simulink model "dynamic_model_euler_with_s"  (R2021b)
settings: Solver=FixedStepAuto  StartTime=0.0  StopTime=simTime  FixedStep=sim_dt  RelTol=1e-3
undefined symbols (not defined in the file): d, g, J_platf, m_mass, m_platf, p, q0, roff, sim_dt, tau, umax, w0
libraries: matrix_library x1
settings Model: SimulationMode=accelerator  Creator=piszy  LastModifiedBy=krzysztof
settings SolverCC: ZeroCrossControl=DisableAll  AlgebraicLoopSolver=TrustRegion
settings DataIOCC: SaveOutput=off  SaveTime=off
settings OptimizationCC: BlockReduction=off  DefaultParameterBehavior=Inlined  BufferReuse=off
settings ModelReferenceCC: ModelReferenceNumInstancesAllowed=Single
settings SFSimCC: CustomCodeUndefinedFunction=UseInterfaceOnly
settings GRTTargetCC: CombineOutputUpdateFcns=off  MatFileLogging=off

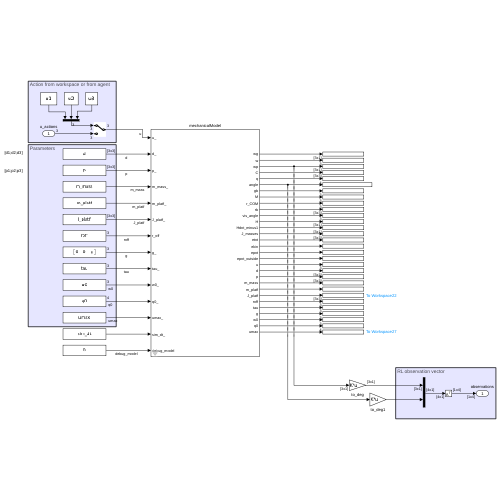
[thumbnail: Simulink's stored preview of the top-level diagram]
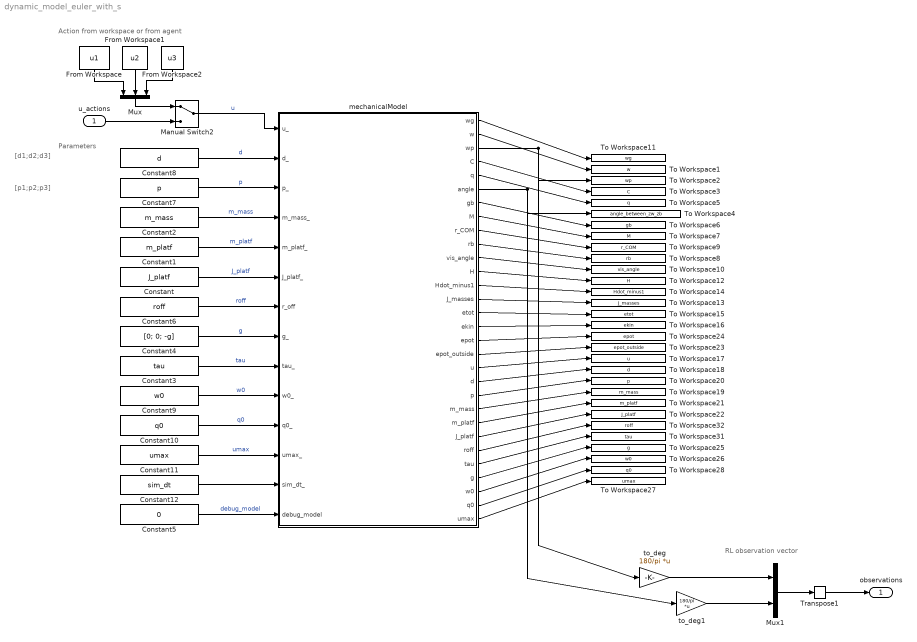
== system dynamic_model_euler_with_s ==
  note: Parameters
  note: Action from workspace or from agent
  note: RL observation vector
  note: [p1;p2;p3]
  note: [d1;d2;d3]
  u_actions : Inport  PortDimensions=[3]
  Constant : Constant  Value=J_platf
  Constant1 : Constant  Value=m_platf
  Constant10 : Constant  Value=q0
  Constant11 : Constant  Value=umax
  Constant12 : Constant  Value=sim_dt
  Constant2 : Constant  Value=m_mass
  Constant3 : Constant  Value=tau
  Constant4 : Constant  Value=[0; 0; -g]
  Constant5 : Constant  Value=0
  Constant6 : Constant  Value=roff
  Constant7 : Constant  Value=p
  Constant8 : Constant  Value=d
  Constant9 : Constant  Value=w0
  From Workspace : FromWorkspace  VariableName=u1
  From Workspace1 : FromWorkspace  VariableName=u2
  From Workspace2 : FromWorkspace  VariableName=u3
  Manual Switch2 : ManualSwitch
  Mux : Mux  Inputs=3
  Mux1 : Mux  Inputs=2
  To Workspace1 : ToWorkspace  VariableName=w  SampleTime=-1
  To Workspace10 : ToWorkspace  VariableName=vis_angle  SampleTime=-1
  To Workspace11 : ToWorkspace  VariableName=wg  SampleTime=-1
  To Workspace12 : ToWorkspace  VariableName=H  SampleTime=-1
  To Workspace13 : ToWorkspace  VariableName=J_masses  SampleTime=-1
  To Workspace14 : ToWorkspace  VariableName=Hdot_minus1  SampleTime=-1
  To Workspace15 : ToWorkspace  VariableName=etot  SampleTime=-1
  To Workspace16 : ToWorkspace  VariableName=ekin  SampleTime=-1
  To Workspace17 : ToWorkspace  VariableName=u  SampleTime=-1
  To Workspace18 : ToWorkspace  VariableName=d  SampleTime=-1
  To Workspace19 : ToWorkspace  VariableName=m_mass  SampleTime=-1
  To Workspace2 : ToWorkspace  VariableName=wp  SampleTime=-1
  To Workspace20 : ToWorkspace  VariableName=p  SampleTime=-1
  To Workspace21 : ToWorkspace  VariableName=m_platf  SampleTime=-1
  To Workspace22 : ToWorkspace  VariableName=J_platf  SampleTime=-1
  To Workspace23 : ToWorkspace  VariableName=epot_outside  SampleTime=-1
  To Workspace24 : ToWorkspace  VariableName=epot  SampleTime=-1
  To Workspace25 : ToWorkspace  VariableName=g  SampleTime=-1
  To Workspace26 : ToWorkspace  VariableName=w0  SampleTime=-1
  To Workspace27 : ToWorkspace  VariableName=umax  SampleTime=-1
  To Workspace28 : ToWorkspace  VariableName=q0  SampleTime=-1
  To Workspace3 : ToWorkspace  VariableName=C  SampleTime=-1
  To Workspace31 : ToWorkspace  VariableName=tau  SampleTime=-1
  To Workspace32 : ToWorkspace  VariableName=roff  SampleTime=-1
  To Workspace4 : ToWorkspace  VariableName=angle_between_zw_zb  SampleTime=-1
  To Workspace5 : ToWorkspace  VariableName=q  SampleTime=-1
  To Workspace6 : ToWorkspace  VariableName=gb  SampleTime=-1
  To Workspace7 : ToWorkspace  VariableName=M  SampleTime=-1
  To Workspace8 : ToWorkspace  VariableName=rb  SampleTime=-1
  To Workspace9 : ToWorkspace  VariableName=r_COM  SampleTime=-1
  Transpose1 : matrix_library/Transpose
      settings: SourceProductBaseCode=SL
  mechanicalModel : Subsystem
      mask help: Simulink:masks:GenSFuncDesc_MD
      mask Help: eval('feval(''rtwprivate'',''rtwhelpview'',''rtw_sfcn_block'')');
  to_deg : Gain  Gain=180/pi  Multiplication=Matrix(K*u)
  to_deg1 : Gain  Gain=180/pi  Multiplication=Matrix(K*u)
  observations : Outport
  wires:
  From Workspace/1 -> Mux/1
  From Workspace1/1 -> Mux/2
  From Workspace2/1 -> Mux/3
  Mux/1 -> Manual Switch2/1
  Manual Switch2/1 -> mechanicalModel/1(u_)  "u"
  u_actions/1 -> Manual Switch2/2
  Mux1/1 -> Transpose1/1
  Transpose1/1 -> observations/1
  Constant2/1 -> mechanicalModel/4(m_mass_)  "m_mass"
  Constant5/1 -> mechanicalModel/14(debug_model)  "debug_model"
  Constant8/1 -> mechanicalModel/2(d_)  "d"
  Constant7/1 -> mechanicalModel/3(p_)  "p"
  Constant1/1 -> mechanicalModel/5(m_platf_)  "m_platf"
  Constant3/1 -> mechanicalModel/9(tau_)  "tau"
  Constant6/1 -> mechanicalModel/7(r_off)  "roff"
  Constant4/1 -> mechanicalModel/8(g_)  "g"
  Constant/1 -> mechanicalModel/6(J_platf_)  "J_platf"
  mechanicalModel/6(angle) -> to_deg1/1, To Workspace4/1
  mechanicalModel/3(wp) -> to_deg/1, To Workspace2/1
  to_deg/1 -> Mux1/1
  to_deg1/1 -> Mux1/2
  Constant9/1 -> mechanicalModel/10(w0_)  "w0"
  Constant10/1 -> mechanicalModel/11(q0_)  "q0"
  Constant11/1 -> mechanicalModel/12(umax_)  "umax"
  Constant12/1 -> mechanicalModel/13(sim_dt_)
  mechanicalModel/1(wg) -> To Workspace11/1
  mechanicalModel/2(w) -> To Workspace1/1
  mechanicalModel/4(C) -> To Workspace3/1
  mechanicalModel/5(q) -> To Workspace5/1
  mechanicalModel/7(gb) -> To Workspace6/1
  mechanicalModel/8(M) -> To Workspace7/1
  mechanicalModel/9(r_COM) -> To Workspace9/1
  mechanicalModel/10(rb) -> To Workspace8/1
  mechanicalModel/11(vis_angle) -> To Workspace10/1
  mechanicalModel/12(H) -> To Workspace12/1
  mechanicalModel/13(Hdot_minus1) -> To Workspace14/1
  mechanicalModel/14(J_masses) -> To Workspace13/1
  mechanicalModel/15(etot) -> To Workspace15/1
  mechanicalModel/16(ekin) -> To Workspace16/1
  mechanicalModel/17(epot) -> To Workspace24/1
  mechanicalModel/18(epot_outside) -> To Workspace23/1
  mechanicalModel/19(u) -> To Workspace17/1
  mechanicalModel/20(d) -> To Workspace18/1
  mechanicalModel/21(p) -> To Workspace20/1
  mechanicalModel/22(m_mass) -> To Workspace19/1
  mechanicalModel/23(m_platf) -> To Workspace21/1
  mechanicalModel/24(J_platf) -> To Workspace22/1
  mechanicalModel/25(roff) -> To Workspace32/1
  mechanicalModel/26(tau) -> To Workspace31/1
  mechanicalModel/27(g) -> To Workspace25/1
  mechanicalModel/28(w0) -> To Workspace26/1
  mechanicalModel/29(q0) -> To Workspace28/1
  mechanicalModel/30(umax) -> To Workspace27/1

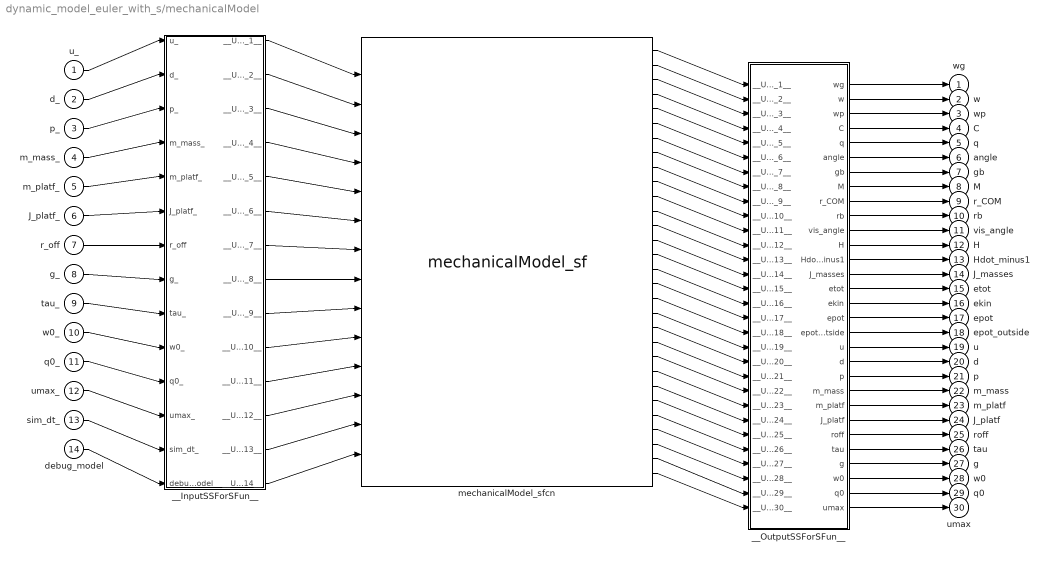
== system dynamic_model_euler_with_s/mechanicalModel ==
  u_ : Inport
  d_ : Inport  Port=2
  p_ : Inport  Port=3
  m_mass_ : Inport  Port=4
  m_platf_ : Inport  Port=5
  J_platf_ : Inport  Port=6
  r_off : Inport  Port=7
  g_ : Inport  Port=8
  tau_ : Inport  Port=9
  w0_ : Inport  Port=10
  q0_ : Inport  Port=11
  umax_ : Inport  Port=12
  sim_dt_ : Inport  Port=13
  debug_model : Inport  Port=14
  __InputSSForSFun__ : Subsystem
  __OutputSSForSFun__ : Subsystem
  mechanicalModel_sfcn : S-Function  FunctionName=mechanicalModel_sf  SFunctionModules=""  SFunctionDeploymentMode=off  EnableBusSupport=off  mask{rtw_sf_name=mechanicalModel_sf, showVar=off}
      mask prompts: rtw_sf_name "Simulink:masks:GenSFuncName_MP"; showVar "Simulink:masks:GenSFuncShowModuleList_MP"
      mask help: Simulink:masks:GenSFuncDesc_MD
      mask init:
      | displist = '';
      | if ~strcmp(get_param(gcb, 'FunctionName'), rtw_sf_name);
      |   set_param(gcb, 'FunctionName', rtw_sf_name);
      | end
      | % Check if we are generating code
      | rtw_mode = false;
      | if strcmpi(get_param(bdroot(gcb),'SimulationStatus'),'Initializing')
      | 	rtw_mode = strcmpi(get_param(bdroot(gcb),'BuildingRTWCode'),'on') && ...
      | 		~strcmpi(get_param(bdroot(gcb),'TargetStyle'),'SimulationTarget');
      | end
      | if showVar || rtw_mode
      | 	if exist('rtwsfunc') == 2 | exist('rtwsfunc') == 6
      | 		tmplist = rtwsfunc(rtw_sf_name,gcb);
      | 		tmplist = DAStudio.message('Simulink:masks:GenSFuncListOfModules_IC', tmplist);
      | 	elseif showVar
      | 		tmplist1 = DAStudio.message('Simulink:masks:GenSFuncListOfModules_IC', '');
      |         tmplist2 = DAStudio.message('Simulink:masks:GenSFuncNotLicensed_IC');
      |         tmplist = [tmplist1 tmplist2];
      |  	end
      | end
      | if showVar
      |   displist = tmplist;
      | end
      settings: CopyFcn=|
      | if ~strcmp(get_param(gcb,'Linkstatus'),'none') && ...
      | ~strcmp(get_param(gcb,'Linkstatus'),'implicit')
      |   set_param(gcb,'LinkStatus','none');
      | end
      mask Help: eval('feval(''rtwprivate'',''rtwhelpview'',''rtw_sfcn_block'')');
      mask Display:
      | port_label('input',1,'u_');
      | port_label('input',2,'d_');
      | port_label('input',3,'p_');
      | port_label('input',4,'m_mass_');
      | port_label('input',5,'m_platf_');
      | port_label('input',6,'J_platf_');
      | port_label('input',7,'r_off');
      | port_label('input',8,'g_');
      | port_label('input',9,'tau_');
      | port_label('input',10,'w0_');
      | port_label('input',11,'q0_');
      | port_label('input',12,'umax_');
      | port_label('input',13,'sim_dt_');
      | port_label('input',14,'debug_model');
      | port_label('output',1,'wg');
      | port_label('output',2,'w');
      | port_label('output',3,'wp');
      | port_label('output',4,'C');
      | port_label('output',5,'q');
      | port_label('output',6,'angle');
      | port_label('output',7,'gb');
      | port_label('output',8,'M');
      | port_label('output',9,'r_COM');
      | port_label('output',10,'rb');
      | port_label('output',11,'vis_angle');
      | port_label('output',12,'H');
      | port_label('output',13,'Hdot_minus1');
      | port_label('output',14,'J_masses');
      | port_label('output',15,'etot');
      | port_label('output',16,'ekin');
      | port_label('output',17,'epot');
      | port_label('output',18,'epot_outside');
      | port_label('output',19,'u');
      | port_label('output',20,'d');
      | port_label('output',21,'p');
      | port_label('output',22,'m_mass');
      | port_label('output',23,'m_platf');
      | port_label('output',24,'J_platf');
      | port_label('output',25,'roff');
      | port_label('output',26,'tau');
      | port_label('output',27,'g');
      | port_label('output',28,'w0');
      | port_label('output',29,'q0');
      | port_label('output',30,'umax');
  wg : Outport
  w : Outport  Port=2
  wp : Outport  Port=3
  C : Outport  Port=4
  q : Outport  Port=5
  angle : Outport  Port=6
  gb : Outport  Port=7
  M : Outport  Port=8
  r_COM : Outport  Port=9
  rb : Outport  Port=10
  vis_angle : Outport  Port=11
  H : Outport  Port=12
  Hdot_minus1 : Outport  Port=13
  J_masses : Outport  Port=14
  etot : Outport  Port=15
  ekin : Outport  Port=16
  epot : Outport  Port=17
  epot_outside : Outport  Port=18
  u : Outport  Port=19
  d : Outport  Port=20
  p : Outport  Port=21
  m_mass : Outport  Port=22
  m_platf : Outport  Port=23
  J_platf : Outport  Port=24
  roff : Outport  Port=25
  tau : Outport  Port=26
  g : Outport  Port=27
  w0 : Outport  Port=28
  q0 : Outport  Port=29
  umax : Outport  Port=30
  wires:
  __OutputSSForSFun__/30(umax) -> umax/1
  __OutputSSForSFun__/29(q0) -> q0/1
  __OutputSSForSFun__/28(w0) -> w0/1
  __OutputSSForSFun__/27(g) -> g/1
  __OutputSSForSFun__/26(tau) -> tau/1
  __OutputSSForSFun__/25(roff) -> roff/1
  __OutputSSForSFun__/24(J_platf) -> J_platf/1
  __OutputSSForSFun__/23(m_platf) -> m_platf/1
  __OutputSSForSFun__/22(m_mass) -> m_mass/1
  __OutputSSForSFun__/21(p) -> p/1
  __OutputSSForSFun__/20(d) -> d/1
  __OutputSSForSFun__/19(u) -> u/1
  __OutputSSForSFun__/18(epot_outside) -> epot_outside/1
  __OutputSSForSFun__/17(epot) -> epot/1
  __OutputSSForSFun__/16(ekin) -> ekin/1
  __OutputSSForSFun__/15(etot) -> etot/1
  __OutputSSForSFun__/14(J_masses) -> J_masses/1
  __OutputSSForSFun__/13(Hdot_minus1) -> Hdot_minus1/1
  __OutputSSForSFun__/12(H) -> H/1
  __OutputSSForSFun__/11(vis_angle) -> vis_angle/1
  __OutputSSForSFun__/10(rb) -> rb/1
  __OutputSSForSFun__/9(r_COM) -> r_COM/1
  __OutputSSForSFun__/8(M) -> M/1
  __OutputSSForSFun__/7(gb) -> gb/1
  __OutputSSForSFun__/6(angle) -> angle/1
  __OutputSSForSFun__/5(q) -> q/1
  __OutputSSForSFun__/4(C) -> C/1
  __OutputSSForSFun__/3(wp) -> wp/1
  __OutputSSForSFun__/2(w) -> w/1
  __OutputSSForSFun__/1(wg) -> wg/1
  mechanicalModel_sfcn/30 -> __OutputSSForSFun__/30(__UniqueInportName__30__)
  mechanicalModel_sfcn/29 -> __OutputSSForSFun__/29(__UniqueInportName__29__)
  mechanicalModel_sfcn/28 -> __OutputSSForSFun__/28(__UniqueInportName__28__)
  mechanicalModel_sfcn/27 -> __OutputSSForSFun__/27(__UniqueInportName__27__)
  mechanicalModel_sfcn/26 -> __OutputSSForSFun__/26(__UniqueInportName__26__)
  mechanicalModel_sfcn/25 -> __OutputSSForSFun__/25(__UniqueInportName__25__)
  mechanicalModel_sfcn/24 -> __OutputSSForSFun__/24(__UniqueInportName__24__)
  mechanicalModel_sfcn/23 -> __OutputSSForSFun__/23(__UniqueInportName__23__)
  mechanicalModel_sfcn/22 -> __OutputSSForSFun__/22(__UniqueInportName__22__)
  mechanicalModel_sfcn/21 -> __OutputSSForSFun__/21(__UniqueInportName__21__)
  mechanicalModel_sfcn/20 -> __OutputSSForSFun__/20(__UniqueInportName__20__)
  mechanicalModel_sfcn/19 -> __OutputSSForSFun__/19(__UniqueInportName__19__)
  mechanicalModel_sfcn/18 -> __OutputSSForSFun__/18(__UniqueInportName__18__)
  mechanicalModel_sfcn/17 -> __OutputSSForSFun__/17(__UniqueInportName__17__)
  mechanicalModel_sfcn/16 -> __OutputSSForSFun__/16(__UniqueInportName__16__)
  mechanicalModel_sfcn/15 -> __OutputSSForSFun__/15(__UniqueInportName__15__)
  mechanicalModel_sfcn/14 -> __OutputSSForSFun__/14(__UniqueInportName__14__)
  mechanicalModel_sfcn/13 -> __OutputSSForSFun__/13(__UniqueInportName__13__)
  mechanicalModel_sfcn/12 -> __OutputSSForSFun__/12(__UniqueInportName__12__)
  mechanicalModel_sfcn/11 -> __OutputSSForSFun__/11(__UniqueInportName__11__)
  mechanicalModel_sfcn/10 -> __OutputSSForSFun__/10(__UniqueInportName__10__)
  mechanicalModel_sfcn/9 -> __OutputSSForSFun__/9(__UniqueInportName__9__)
  mechanicalModel_sfcn/8 -> __OutputSSForSFun__/8(__UniqueInportName__8__)
  mechanicalModel_sfcn/7 -> __OutputSSForSFun__/7(__UniqueInportName__7__)
  mechanicalModel_sfcn/6 -> __OutputSSForSFun__/6(__UniqueInportName__6__)
  mechanicalModel_sfcn/5 -> __OutputSSForSFun__/5(__UniqueInportName__5__)
  mechanicalModel_sfcn/4 -> __OutputSSForSFun__/4(__UniqueInportName__4__)
  mechanicalModel_sfcn/3 -> __OutputSSForSFun__/3(__UniqueInportName__3__)
  mechanicalModel_sfcn/2 -> __OutputSSForSFun__/2(__UniqueInportName__2__)
  mechanicalModel_sfcn/1 -> __OutputSSForSFun__/1(__UniqueInportName__1__)
  __InputSSForSFun__/14(__UniqueOutportName__14__) -> mechanicalModel_sfcn/14
  __InputSSForSFun__/13(__UniqueOutportName__13__) -> mechanicalModel_sfcn/13
  __InputSSForSFun__/12(__UniqueOutportName__12__) -> mechanicalModel_sfcn/12
  __InputSSForSFun__/11(__UniqueOutportName__11__) -> mechanicalModel_sfcn/11
  __InputSSForSFun__/10(__UniqueOutportName__10__) -> mechanicalModel_sfcn/10
  __InputSSForSFun__/9(__UniqueOutportName__9__) -> mechanicalModel_sfcn/9
  __InputSSForSFun__/8(__UniqueOutportName__8__) -> mechanicalModel_sfcn/8
  __InputSSForSFun__/7(__UniqueOutportName__7__) -> mechanicalModel_sfcn/7
  __InputSSForSFun__/6(__UniqueOutportName__6__) -> mechanicalModel_sfcn/6
  __InputSSForSFun__/5(__UniqueOutportName__5__) -> mechanicalModel_sfcn/5
  __InputSSForSFun__/4(__UniqueOutportName__4__) -> mechanicalModel_sfcn/4
  __InputSSForSFun__/3(__UniqueOutportName__3__) -> mechanicalModel_sfcn/3
  __InputSSForSFun__/2(__UniqueOutportName__2__) -> mechanicalModel_sfcn/2
  __InputSSForSFun__/1(__UniqueOutportName__1__) -> mechanicalModel_sfcn/1
  debug_model/1 -> __InputSSForSFun__/14(debug_model)
  sim_dt_/1 -> __InputSSForSFun__/13(sim_dt_)
  umax_/1 -> __InputSSForSFun__/12(umax_)
  q0_/1 -> __InputSSForSFun__/11(q0_)
  w0_/1 -> __InputSSForSFun__/10(w0_)
  tau_/1 -> __InputSSForSFun__/9(tau_)
  g_/1 -> __InputSSForSFun__/8(g_)
  r_off/1 -> __InputSSForSFun__/7(r_off)
  J_platf_/1 -> __InputSSForSFun__/6(J_platf_)
  m_platf_/1 -> __InputSSForSFun__/5(m_platf_)
  m_mass_/1 -> __InputSSForSFun__/4(m_mass_)
  p_/1 -> __InputSSForSFun__/3(p_)
  d_/1 -> __InputSSForSFun__/2(d_)
  u_/1 -> __InputSSForSFun__/1(u_)

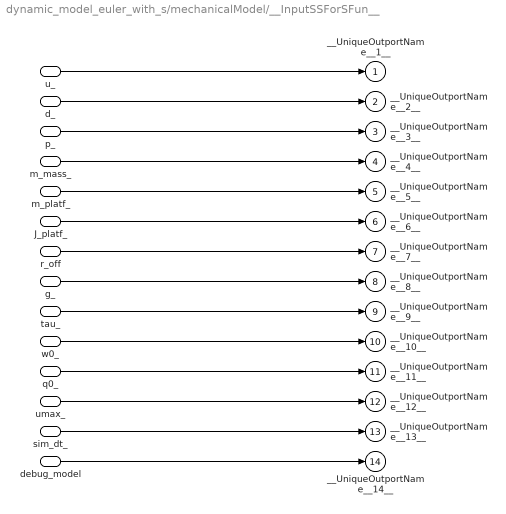
== system dynamic_model_euler_with_s/mechanicalModel/__InputSSForSFun__ ==
  u_ : Inport
  d_ : Inport  Port=2
  p_ : Inport  Port=3
  m_mass_ : Inport  Port=4
  m_platf_ : Inport  Port=5
  J_platf_ : Inport  Port=6
  r_off : Inport  Port=7
  g_ : Inport  Port=8
  tau_ : Inport  Port=9
  w0_ : Inport  Port=10
  q0_ : Inport  Port=11
  umax_ : Inport  Port=12
  sim_dt_ : Inport  Port=13
  debug_model : Inport  Port=14
  __UniqueOutportName__1__ : Outport
  __UniqueOutportName__2__ : Outport  Port=2
  __UniqueOutportName__3__ : Outport  Port=3
  __UniqueOutportName__4__ : Outport  Port=4
  __UniqueOutportName__5__ : Outport  Port=5
  __UniqueOutportName__6__ : Outport  Port=6
  __UniqueOutportName__7__ : Outport  Port=7
  __UniqueOutportName__8__ : Outport  Port=8
  __UniqueOutportName__9__ : Outport  Port=9
  __UniqueOutportName__10__ : Outport  Port=10
  __UniqueOutportName__11__ : Outport  Port=11
  __UniqueOutportName__12__ : Outport  Port=12
  __UniqueOutportName__13__ : Outport  Port=13
  __UniqueOutportName__14__ : Outport  Port=14
  wires:
  debug_model/1 -> __UniqueOutportName__14__/1
  sim_dt_/1 -> __UniqueOutportName__13__/1
  umax_/1 -> __UniqueOutportName__12__/1
  q0_/1 -> __UniqueOutportName__11__/1
  w0_/1 -> __UniqueOutportName__10__/1
  tau_/1 -> __UniqueOutportName__9__/1
  g_/1 -> __UniqueOutportName__8__/1
  r_off/1 -> __UniqueOutportName__7__/1
  J_platf_/1 -> __UniqueOutportName__6__/1
  m_platf_/1 -> __UniqueOutportName__5__/1
  m_mass_/1 -> __UniqueOutportName__4__/1
  p_/1 -> __UniqueOutportName__3__/1
  d_/1 -> __UniqueOutportName__2__/1
  u_/1 -> __UniqueOutportName__1__/1

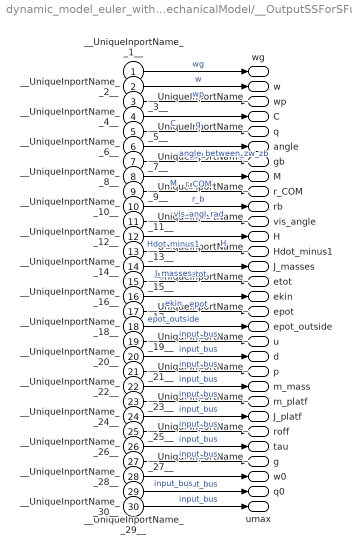
== system dynamic_model_euler_with_s/mechanicalModel/__OutputSSForSFun__ ==
  __UniqueInportName__1__ : Inport
  __UniqueInportName__2__ : Inport  Port=2
  __UniqueInportName__3__ : Inport  Port=3
  __UniqueInportName__4__ : Inport  Port=4
  __UniqueInportName__5__ : Inport  Port=5
  __UniqueInportName__6__ : Inport  Port=6
  __UniqueInportName__7__ : Inport  Port=7
  __UniqueInportName__8__ : Inport  Port=8
  __UniqueInportName__9__ : Inport  Port=9
  __UniqueInportName__10__ : Inport  Port=10
  __UniqueInportName__11__ : Inport  Port=11
  __UniqueInportName__12__ : Inport  Port=12
  __UniqueInportName__13__ : Inport  Port=13
  __UniqueInportName__14__ : Inport  Port=14
  __UniqueInportName__15__ : Inport  Port=15
  __UniqueInportName__16__ : Inport  Port=16
  __UniqueInportName__17__ : Inport  Port=17
  __UniqueInportName__18__ : Inport  Port=18
  __UniqueInportName__19__ : Inport  Port=19
  __UniqueInportName__20__ : Inport  Port=20
  __UniqueInportName__21__ : Inport  Port=21
  __UniqueInportName__22__ : Inport  Port=22
  __UniqueInportName__23__ : Inport  Port=23
  __UniqueInportName__24__ : Inport  Port=24
  __UniqueInportName__25__ : Inport  Port=25
  __UniqueInportName__26__ : Inport  Port=26
  __UniqueInportName__27__ : Inport  Port=27
  __UniqueInportName__28__ : Inport  Port=28
  __UniqueInportName__29__ : Inport  Port=29
  __UniqueInportName__30__ : Inport  Port=30
  wg : Outport
  w : Outport  Port=2
  wp : Outport  Port=3
  C : Outport  Port=4
  q : Outport  Port=5
  angle : Outport  Port=6
  gb : Outport  Port=7
  M : Outport  Port=8
  r_COM : Outport  Port=9
  rb : Outport  Port=10
  vis_angle : Outport  Port=11
  H : Outport  Port=12
  Hdot_minus1 : Outport  Port=13
  J_masses : Outport  Port=14
  etot : Outport  Port=15
  ekin : Outport  Port=16
  epot : Outport  Port=17
  epot_outside : Outport  Port=18
  u : Outport  Port=19
  d : Outport  Port=20
  p : Outport  Port=21
  m_mass : Outport  Port=22
  m_platf : Outport  Port=23
  J_platf : Outport  Port=24
  roff : Outport  Port=25
  tau : Outport  Port=26
  g : Outport  Port=27
  w0 : Outport  Port=28
  q0 : Outport  Port=29
  umax : Outport  Port=30
  wires:
  __UniqueInportName__30__/1 -> umax/1  "input_bus"
  __UniqueInportName__29__/1 -> q0/1  "input_bus"
  __UniqueInportName__28__/1 -> w0/1  "input_bus"
  __UniqueInportName__27__/1 -> g/1  "input_bus"
  __UniqueInportName__26__/1 -> tau/1  "input_bus"
  __UniqueInportName__25__/1 -> roff/1  "input_bus"
  __UniqueInportName__24__/1 -> J_platf/1  "input_bus"
  __UniqueInportName__23__/1 -> m_platf/1  "input_bus"
  __UniqueInportName__22__/1 -> m_mass/1  "input_bus"
  __UniqueInportName__21__/1 -> p/1  "input_bus"
  __UniqueInportName__20__/1 -> d/1  "input_bus"
  __UniqueInportName__19__/1 -> u/1  "input_bus"
  __UniqueInportName__18__/1 -> epot_outside/1  "epot_outside"
  __UniqueInportName__17__/1 -> epot/1  "epot"
  __UniqueInportName__16__/1 -> ekin/1  "ekin"
  __UniqueInportName__15__/1 -> etot/1  "etot"
  __UniqueInportName__14__/1 -> J_masses/1  "J_masses"
  __UniqueInportName__13__/1 -> Hdot_minus1/1  "Hdot_minus1"
  __UniqueInportName__12__/1 -> H/1  "H"
  __UniqueInportName__11__/1 -> vis_angle/1  "vis_angl_rad"
  __UniqueInportName__10__/1 -> rb/1  "r_b"
  __UniqueInportName__9__/1 -> r_COM/1  "r_COM"
  __UniqueInportName__8__/1 -> M/1  "M"
  __UniqueInportName__7__/1 -> gb/1  "gb"
  __UniqueInportName__6__/1 -> angle/1  "angle_between_zw_zb"
  __UniqueInportName__5__/1 -> q/1  "q"
  __UniqueInportName__4__/1 -> C/1  "C"
  __UniqueInportName__3__/1 -> wp/1  "wp"
  __UniqueInportName__2__/1 -> w/1  "w"
  __UniqueInportName__1__/1 -> wg/1  "wg"
